simulink model "OperatingModeAndErrorLogic_Dashboard"  (R2024b)
settings: Solver=VariableStepAuto  StartTime=0.0  StopTime=inf  RelTol=1e-3
undefined symbols (not defined in the file): operatingMode
libraries: simulink x1
settings Model: Creator=vlenzi  LastModifiedBy=vlenzi
settings DebuggingCC: ParameterPrecisionLossMsg=none
settings RTWCC: GPUComputeCapability=3.5
settings ConfigComp: CovEnable=on  RecordCoverage=on  CovModelRefEnable=on

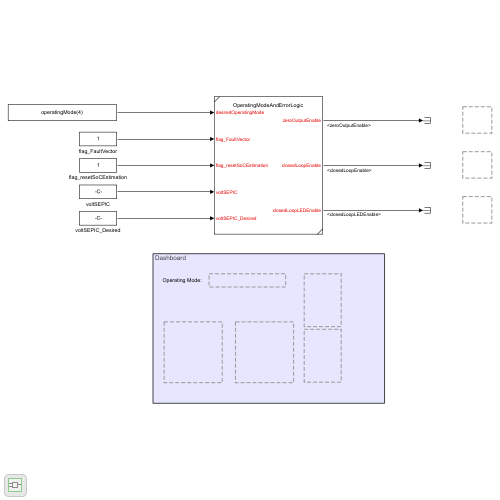
[thumbnail: Simulink's stored preview of the top-level diagram]
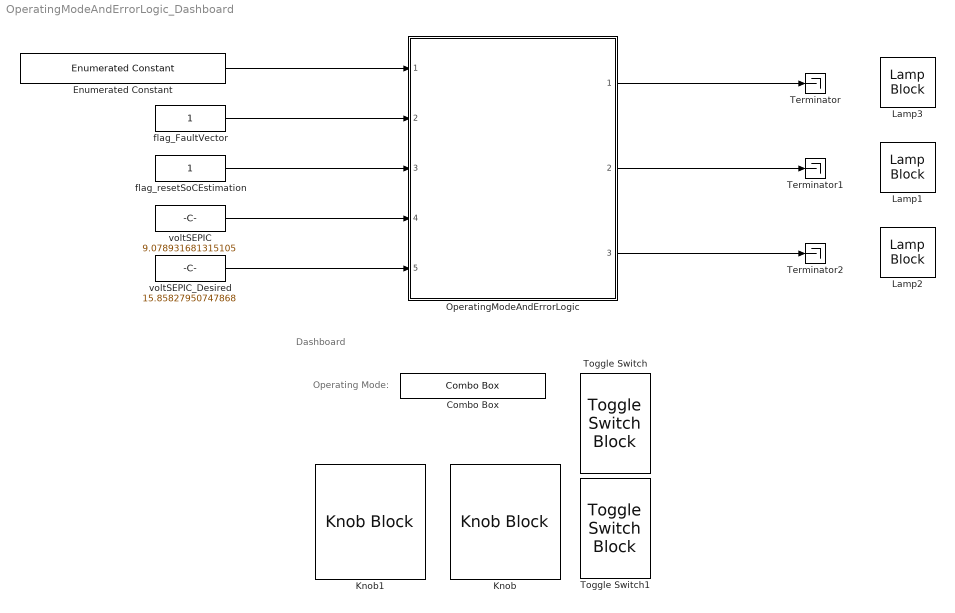
== system OperatingModeAndErrorLogic_Dashboard ==
  note: Operating Mode:
  note: Dashboard
  Combo Box : ComboBox  LabelPosition=Hide  SelectedLabel=AllClosedLoop  UseEnumeratedDataType=on  EnumeratedDataType=operatingMode
      settings: Values={{'NoOutput', 'AllOpenLoop', 'VoltOpen_CurrClosed', 'VoltClosed_CurrOpen', 'AllClosedLoop', 'AutomaticOperation'}, [0 1 2 3 4 5]}
  Enumerated Constant : simulink/Sources/Enumerated Constant  OutDataTypeStr=Enum:operatingMode  Value=operatingMode(4)  SampleTime=-1
  Knob : KnobBlock  ScaleMax=20
  Knob1 : KnobBlock  ScaleMax=20
  Lamp1 : LampBlock  LabelPosition=Hide
  Lamp2 : LampBlock  LabelPosition=Hide
  Lamp3 : LampBlock  LabelPosition=Hide
  OperatingModeAndErrorLogic : Subsystem  ReferencedSubsystem=OperatingModeAndErrorLogic
  Terminator : Terminator
  Terminator1 : Terminator
  Terminator2 : Terminator
  Toggle Switch : ToggleSwitchBlock
      settings: Values={{'Off', 'On'}, [0 1]}
  Toggle Switch1 : ToggleSwitchBlock
      settings: Values={{'Off', 'On'}, [0 1]}
  flag_FaultVector : Constant  OutDataTypeStr=boolean
  flag_resetSoCEstimation : Constant  OutDataTypeStr=boolean
  voltSEPIC : Constant  Value=9.078931681315105  OutDataTypeStr=single
  voltSEPIC_Desired : Constant  Value=15.85827950747868  OutDataTypeStr=single
  wires:
  OperatingModeAndErrorLogic/1 -> Terminator/1
  OperatingModeAndErrorLogic/2 -> Terminator1/1
  OperatingModeAndErrorLogic/3 -> Terminator2/1
  Enumerated Constant/1 -> OperatingModeAndErrorLogic/1
  flag_FaultVector/1 -> OperatingModeAndErrorLogic/2
  flag_resetSoCEstimation/1 -> OperatingModeAndErrorLogic/3
  voltSEPIC/1 -> OperatingModeAndErrorLogic/4
  voltSEPIC_Desired/1 -> OperatingModeAndErrorLogic/5
